simulink model "bmssoftware"  (R2018a)
settings: Solver=FixedStepDiscrete  StartTime=0.0  StopTime=10.0  FixedStep=0.1  RelTol=1e-3  EnableMultiTasking=on
undefined symbols (not defined in the file or in its folder): MaxlimtVolt, MinlimtVolt
settings Model: DataDictionary=data.sldd  Creator=胡桐  LastModifiedBy=胡桐
settings SolverCC: AutoInsertRateTranBlk=on
settings DataIOCC: LimitDataPoints=on
settings OptimizationCC: LifeSpan=inf
settings DebuggingCC: AllowSymbolicDim=off  SFUnexpectedBacktrackingDiag=warning  SFNoUnconditionalDefaultTransitionDiag=warning  SFExecutionAtInitializationDiag=none
settings CodeAppCC: StateflowObjectComments=on
settings GRTTargetCC: TargetLangStandard=C89/C90 (ANSI)  GeneratePreprocessorConditionals=Disable all
settings ConfigComp: CovMetricSettings=dw  CovHtmlReporting=on  CovSaveCumulativeToWorkspaceVar=on  CovSaveSingleToWorkspaceVar=on  CovShowResultsExplorer=off  CovExternalEMLEnable=off  CovSFcnEnable=off

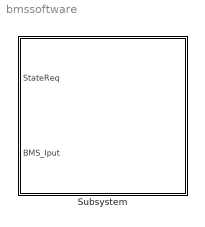
== system bmssoftware ==
  Subsystem : Subsystem

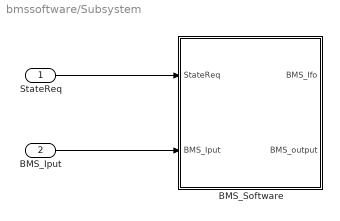
== system bmssoftware/Subsystem ==
  StateReq : Inport  OutDataTypeStr=single
  BMS_Iput : Inport  Port=2  OutDataTypeStr=single
  BMS_Software : Subsystem
  wires:
  BMS_Iput/1 -> BMS_Software/2(BMS_Iput)
  StateReq/1 -> BMS_Software/1(StateReq)

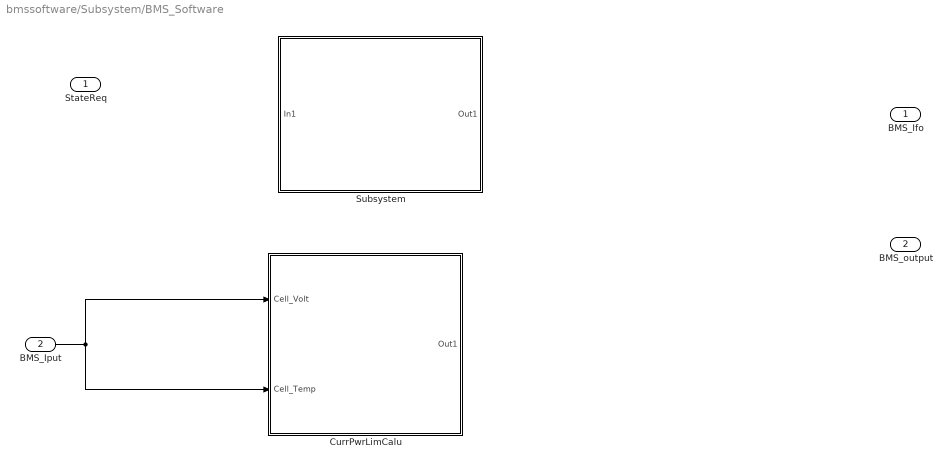
== system bmssoftware/Subsystem/BMS_Software ==
  StateReq : Inport
  BMS_Iput : Inport  Port=2
  CurrPwrLimCalu : Subsystem
  Subsystem : Subsystem
  BMS_Ifo : Outport
  BMS_output : Outport  Port=2
  wires:
  BMS_Iput/1 -> CurrPwrLimCalu/2(Cell_Temp), CurrPwrLimCalu/1(Cell_Volt)

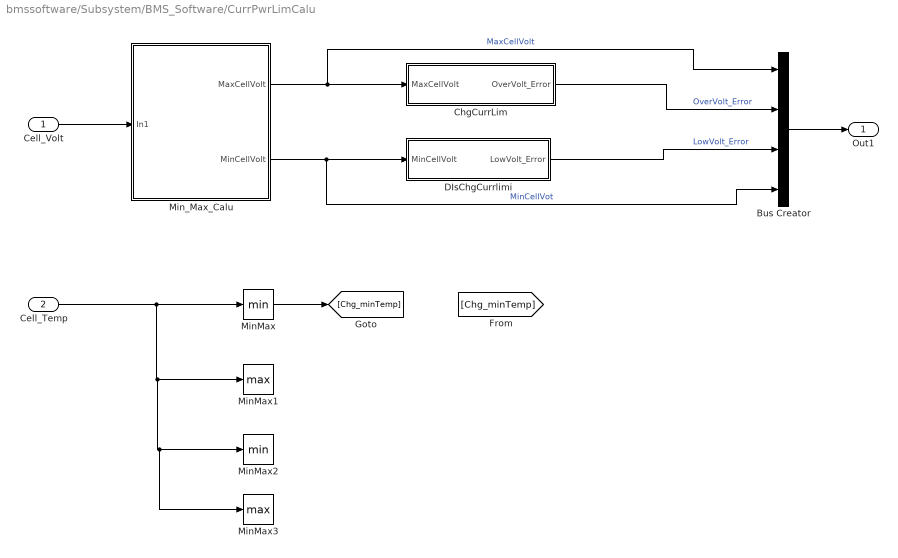
== system bmssoftware/Subsystem/BMS_Software/CurrPwrLimCalu ==
  Cell_Volt : Inport
  Cell_Temp : Inport  Port=2
  Bus Creator : BusCreator  Inputs=4
  ChgCurrLim : Subsystem
  DIsChgCurrlimi : Subsystem
  MinMax : MinMax
  MinMax1 : MinMax  Function=max
  MinMax2 : MinMax
  MinMax3 : MinMax  Function=max
  Min_Max_Calu : Subsystem
  Out1 : Outport
  wires:
  Cell_Volt/1 -> Min_Max_Calu/1(In1)
  Min_Max_Calu/1(MaxCellVolt) -> Bus Creator/1, ChgCurrLim/1(MaxCellVolt)  "MaxCellVolt"
  Min_Max_Calu/2(MinCellVolt) -> Bus Creator/4, DIsChgCurrlimi/1(MinCellVolt)  "MinCellVot"
  Cell_Temp/1 -> MinMax3/1, MinMax2/1, MinMax1/1, MinMax/1
  MinMax/1 -> [Chg_minTemp]
  Bus Creator/1 -> Out1/1
  ChgCurrLim/1(OverVolt_Error) -> Bus Creator/2  "OverVolt_Error"
  DIsChgCurrlimi/1(LowVolt_Error) -> Bus Creator/3  "LowVolt_Error"

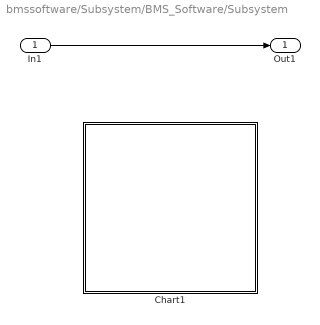
== system bmssoftware/Subsystem/BMS_Software/Subsystem ==
  In1 : Inport
  Chart1 : Stateflow chart  TreatAsAtomicUnit=on
  Out1 : Outport
  wires:
  In1/1 -> Out1/1

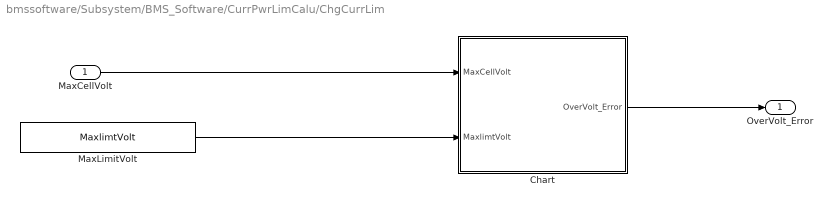
== system bmssoftware/Subsystem/BMS_Software/CurrPwrLimCalu/ChgCurrLim ==
  MaxCellVolt : Inport
  Chart : Stateflow chart  TreatAsAtomicUnit=on
  MaxLimitVolt : Constant  Value=MaxlimtVolt
  OverVolt_Error : Outport
  wires:
  MaxCellVolt/1 -> Chart/1(MaxCellVolt)
  MaxLimitVolt/1 -> Chart/2(MaxlimtVolt)
  Chart/1(OverVolt_Error) -> OverVolt_Error/1

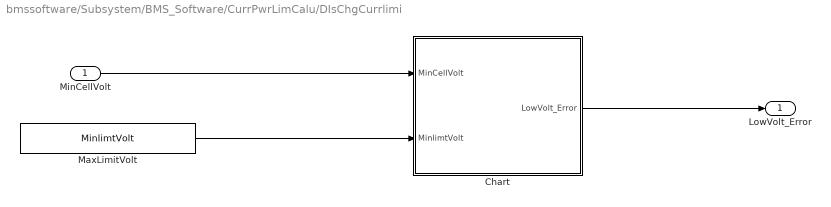
== system bmssoftware/Subsystem/BMS_Software/CurrPwrLimCalu/DIsChgCurrlimi ==
  MinCellVolt : Inport
  Chart : Stateflow chart  TreatAsAtomicUnit=on
  MaxLimitVolt : Constant  Value=MinlimtVolt
  LowVolt_Error : Outport
  wires:
  MaxLimitVolt/1 -> Chart/2(MinlimtVolt)
  MinCellVolt/1 -> Chart/1(MinCellVolt)
  Chart/1(LowVolt_Error) -> LowVolt_Error/1

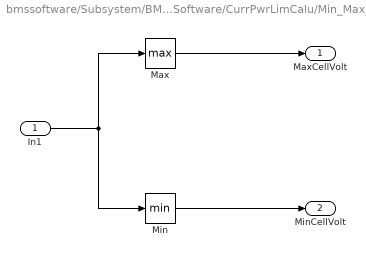
== system bmssoftware/Subsystem/BMS_Software/CurrPwrLimCalu/Min_Max_Calu ==
  In1 : Inport
  Max : MinMax  Function=max
  Min : MinMax
  MaxCellVolt : Outport
  MinCellVolt : Outport  Port=2
  wires:
  In1/1 -> Min/1, Max/1
  Max/1 -> MaxCellVolt/1
  Min/1 -> MinCellVolt/1

== stateflow chart bmssoftware/Subsystem/BMS_Software/Subsystem/Chart1 ==

== stateflow chart bmssoftware/Subsystem/BMS_Software/CurrPwrLimCalu/DIsChgCurrlimi/Chart ==
  state OverVolt
    du:
    LowVolt_Error=1;
  state NomalVolt
    du:
    LowVolt_Error=0;
  (default) -> NomalVolt
  NomalVolt -> OverVolt : [MinCellVolt>MinlimtVolt]{after(2,sec)}
  OverVolt -> NomalVolt
  data: MinCellVolt input; MinlimtVolt input; LowVolt_Error output

== stateflow chart bmssoftware/Subsystem/BMS_Software/CurrPwrLimCalu/ChgCurrLim/Chart ==
  state OverVolt
    du:
    OverVolt_Error=1;
  state NomalVolt
    du:
    OverVolt_Error=0;
  (default) -> NomalVolt
  NomalVolt -> OverVolt : [MaxCellVolt>MaxlimtVolt]{after(2,sec)}
  OverVolt -> NomalVolt
  data: MaxCellVolt input; MaxlimtVolt input; OverVolt_Error output
